simulink subsystem "Vehicle1D_input_refsub"  (R2022a)
settings: Solver=VariableStepAuto  StartTime=0.0  StopTime=10.0  RelTol=1e-3
settings Model: Creator=isaacito  LastModifiedBy=isaacito

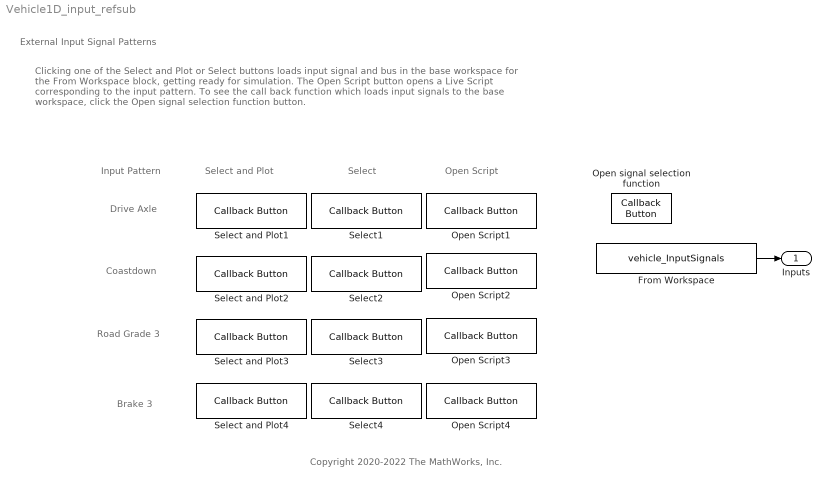
== system Vehicle1D_input_refsub ==
  note: Clicking one of the Select and Plot or Select buttons loads input signal and bus
      | in the base workspace for the From Workspace block, getting ready for simulation.
      | The Open Script button opens a Live Script corresponding to the input pattern.
      | To see the call back function which loads input signals to the base workspace,
      | click the Open signal selection function button.
  note: External Input Signal Patterns
  note: Drive Axle
  note: Coastdown
  note: Road Grade 3
  note: Brake 3
  note: Select and Plot
  note: Select
  note: Copyright 2020-2022 The MathWorks, Inc.
  note: Input Pattern
  note: Open Script
  From Workspace : FromWorkspace  VariableName=vehicle_InputSignals  OutDataTypeStr=Bus: vehicle_InputBus  OutputAfterFinalValue=Holding final value
      settings: AttributesFormatString=|
      | %<OutDataTypeStr>
      | Interpolate: %<Interpolate>
  Open Script{1..4} (4 alike) : CallbackButton  ButtonText=Open Script
      Open Script1 settings: ClickFcn=edit Vehicle1D_testcase_DriveAxle
      Open Script2 settings: ClickFcn=edit Vehicle1D_testcase_Coastdown
      Open Script3 settings: ClickFcn=edit Vehicle1D_testcase_RoadGrade3
      Open Script4 settings: ClickFcn=edit Vehicle1D_testcase_Brake3
  Open signal selection function : CallbackButton  ButtonText=Open
      settings: ClickFcn=edit Vehicle1D_selectInput
  Select and Plot{1..4} (4 alike) : CallbackButton  ButtonText=Select and Plot
      Select and Plot1 settings: ClickFcn=|
      | Vehicle1D_selectInput( ...
      |     InputPattern = "DriveAxle", ...
      |     DisplayMessage = true )
      | 
      | Vehicle1D_plotInputs( ...
      |     "vehicle_InputSignals", ...
      |     WindowName = "Drive Axle");
      Select and Plot2 settings: ClickFcn=|
      | Vehicle1D_selectInput( ...
      |     InputPattern = "Coastdown", ...
      |     DisplayMessage = true )
      | 
      | Vehicle1D_plotInputs( ...
      |     "vehicle_InputSignals", ...
      |     WindowName = "Coastdown");
      Select and Plot3 settings: ClickFcn=|
      | Vehicle1D_selectInput( ...
      |     InputPattern = "RoadGrade3", ...
      |     DisplayMessage = true )
      | 
      | Vehicle1D_plotInputs( ...
      |     "vehicle_InputSignals", ...
      |     WindowName = "Road Grade 3");
      Select and Plot4 settings: ClickFcn=|
      | Vehicle1D_selectInput( ...
      |     InputPattern = "Brake3", ...
      |     DisplayMessage = true )
      | 
      | Vehicle1D_plotInputs( ...
      |     "vehicle_InputSignals", ...
      |     WindowName = "Brake 3");
  Select{1..4} (4 alike) : CallbackButton  ButtonText=Select
      Select1 settings: ClickFcn=|
      | Vehicle1D_selectInput( ...
      |     InputPattern = "DriveAxle", ...
      |     DisplayMessage = true)
      Select2 settings: ClickFcn=|
      | Vehicle1D_selectInput( ...
      |     InputPattern = "Coastdown", ...
      |     DisplayMessage = true)
      Select3 settings: ClickFcn=|
      | Vehicle1D_selectInput( ...
      |     InputPattern = "RoadGrade3", ...
      |     DisplayMessage = true)
      Select4 settings: ClickFcn=|
      | Vehicle1D_selectInput( ...
      |     InputPattern = "Brake3", ...
      |     DisplayMessage = true)
  Inputs : Outport
  wires:
  From Workspace/1 -> Inputs/1
